simulink model "modelGodMac"  (R2019b)
settings: Solver=ode4  StartTime=0.0  StopTime=50  FixedStep=0.01  RelTol=1e-3
values from neighbouring files (symbols this model uses):
  A = [-Ya_Alpha 1 0 ... (first row only)    [StateSpace.m]    (also in matan.m = [1 -1/p; modelGodPrint.m = figure; print2.m = figure)
  B = [0;Mz_deltaB;0]    [StateSpace.m]    (also in matan.m = [0; -K_v*Vzad/(1/(W*Wpriv)+K_wz)]; modelGodPrint.m = figure)
  C = [1 0 0; 0 1 0; 0 0 1]    [StateSpace.m]    (also in modelGodPrint.m = figure)
  D = [0;0;0]    [StateSpace.m]    (also in modelGodPrint.m = figure)
  i_H = 0.8/(1/Ya_Alpha*V)    [Synthesis_of_ACS.m]
  i_p = i_H^2*V    [Synthesis_of_ACS.m]
  K_v = nu*K_wz    [Synthesis_of_ACS.m]
  K_wz = e*K_wzGr    [Synthesis_of_ACS.m]
libraries: cstblocks x2
settings Model: Creator=aleksejpasenko  LastModifiedBy=aleksejpasenko

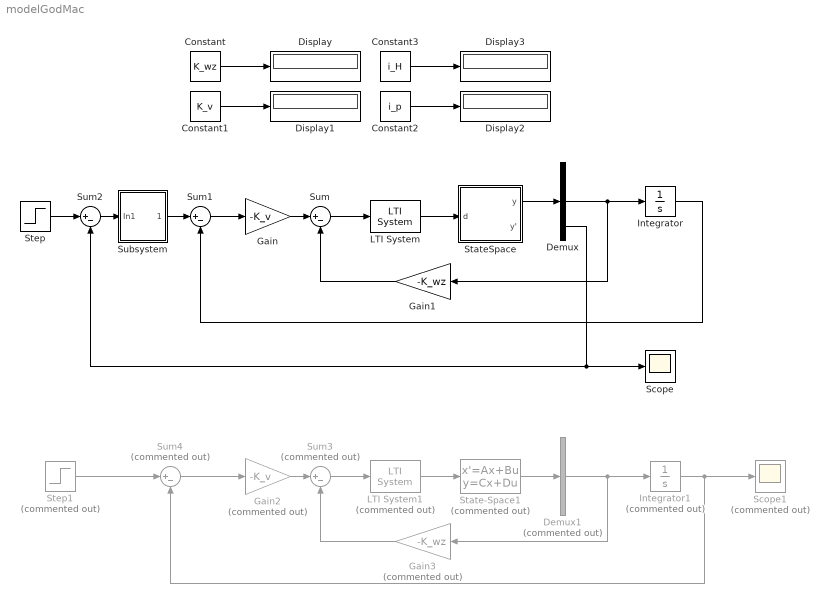
== system modelGodMac ==
  Constant : Constant  Value=K_wz
  Constant1 : Constant  Value=K_v
  Constant2 : Constant  Value=i_p
  Constant3 : Constant  Value=i_H
  Demux : Demux  Outputs=3
  Demux1 : Demux  Commented=on  Outputs=3
  Display{,1..3} (4 alike) : Display
  Gain : Gain  Gain=-K_v
  Gain1 : Gain  Gain=-K_wz
  Gain2 : Gain  Commented=on  Gain=-K_v
  Gain3 : Gain  Commented=on  Gain=-K_wz
  Integrator : Integrator
  Integrator1 : Integrator  Commented=on
  LTI System : cstblocks/LTI System  sys=Drive  IC=[]
  LTI System1 : cstblocks/LTI System  Commented=on  sys=Drive  IC=[]
  Scope : Scope
  Scope1 : Scope  Commented=on
  State-Space1 : StateSpace  Commented=on  A=A  B=B  C=C  D=D  InitialCondition=0
  StateSpace : Subsystem
  Step : Step  SampleTime=0
  Step1 : Step  Commented=on  SampleTime=0
  Subsystem : Subsystem
  Sum : Sum  Inputs=|+-
  Sum1 : Sum  Inputs=|+-
  Sum2 : Sum  Inputs=|+-
  Sum3 : Sum  Commented=on  Inputs=|+-
  Sum4 : Sum  Commented=on  Inputs=|+-
  wires:
  StateSpace/1(y) -> Demux/1
  LTI System/1 -> StateSpace/1(d)
  Gain/1 -> Sum/1
  Demux/2 -> Gain1/1, Integrator/1
  Gain1/1 -> Sum/2
  Sum/1 -> LTI System/1
  Integrator/1 -> Sum1/2
  Sum1/1 -> Gain/1
  Sum2/1 -> Subsystem/1(In1)
  Demux/3 -> Scope/1, Sum2/2
  Subsystem/1(Out1) -> Sum1/1
  Step/1 -> Sum2/1
  LTI System1/1 -> State-Space1/1
  Sum4/1 -> Gain2/1
  Demux1/2 -> Integrator1/1, Gain3/1
  Gain3/1 -> Sum3/2
  Sum3/1 -> LTI System1/1
  State-Space1/1 -> Demux1/1
  Gain2/1 -> Sum3/1
  Integrator1/1 -> Scope1/1, Sum4/2
  Step1/1 -> Sum4/1
  Constant/1 -> Display/1
  Constant1/1 -> Display1/1
  Constant2/1 -> Display2/1
  Constant3/1 -> Display3/1

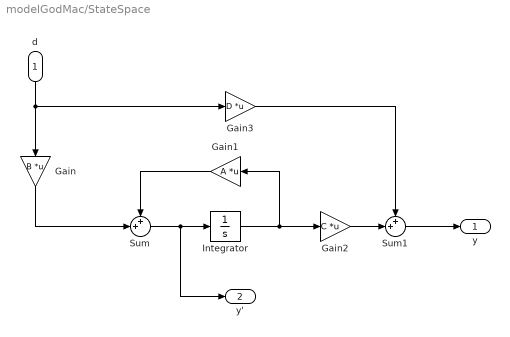
== system modelGodMac/StateSpace ==
  d : Inport
  Gain : Gain  Gain=B  Multiplication=Matrix(K*u)
  Gain1 : Gain  Gain=A  Multiplication=Matrix(K*u)
  Gain2 : Gain  Gain=C  Multiplication=Matrix(K*u)
  Gain3 : Gain  Gain=D  Multiplication=Matrix(K*u)
  Integrator : Integrator
  Sum : Sum  Inputs=++|
  Sum1 : Sum  Inputs=++|
  y : Outport
  y' : Outport  Port=2
  wires:
  d/1 -> Gain3/1, Gain/1
  Gain1/1 -> Sum/1
  Sum/1 -> y'/1, Integrator/1
  Integrator/1 -> Gain1/1, Gain2/1
  Gain2/1 -> Sum1/2
  Sum1/1 -> y/1
  Gain3/1 -> Sum1/1
  Gain/1 -> Sum/2

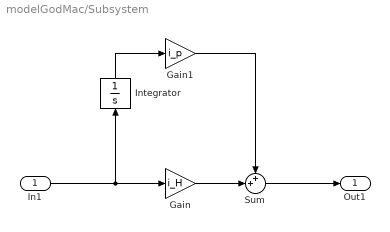
== system modelGodMac/Subsystem ==
  In1 : Inport
  Gain : Gain  Gain=i_H
  Gain1 : Gain  Gain=i_p
  Integrator : Integrator
  Sum : Sum  Inputs=++|
  Out1 : Outport
  wires:
  In1/1 -> Integrator/1, Gain/1
  Sum/1 -> Out1/1
  Gain/1 -> Sum/2
  Integrator/1 -> Gain1/1
  Gain1/1 -> Sum/1
